simulink model "HCS_Sim_r9_final"  (R2023a)
settings: Solver=ode4  StartTime=0.0  StopTime=24  FixedStep=5e-3  RelTol=1e-3  EnableMultiTasking=on
libraries: simulink x26, simulink_extras x11, arduinolib x8, spspowerguiLib x1
(part 5 of 5)

== matlab function HCS_Sim_r9_final/Total Resource Monitor ==
  data: tou input; grid2fly input; fly2grid input; ev_g2v input; grid2station output; ev_v2g input; station2grid output; opCost output; savings output; ev_g2v_cost output size=[1 3]; ev_v2g_cost output size=[1 3]; grid2fly_cost output; fly2grid_cost output; elec_g2v input; elec_v2g input
function [grid2station, station2grid, opCost, savings, ev_g2v_cost, ev_v2g_cost, grid2fly_cost, fly2grid_cost]   = totalResourceMonitor(tou, grid2fly, fly2grid, ev_g2v, ev_v2g,elec_g2v, elec_v2g)
min = 60; % 1 hr in mins
sec = 60; % 1 min in seconds

ev_g2v_delta = zeros(1, 3);
ev_v2g_delta = zeros(1, 3);
ev_g2v_cost = zeros(1, 3);
ev_v2g_cost = zeros(1, 3);
grid2fly_cost = 0;
fly2grid_cost = 0;

% define rates
if tou == 1
    rate = 0.087; % $/kWh --> $/kWs
elseif tou == 3
    rate = 0.122; % $/kWh --> $/kWs
elseif tou == 4
    rate = 0.182; % $/kWh --> $/kWs
elseif tou == 2
    rate = 0.122; % $/kWh --> $/kWs
else
    rate = 0;
end

% define persistents (memory values)
persistent ev_g2v_prev ev_v2g_prev grid2fly_prev fly2grid_prev grid2station_prev station2grid_prev opCost_prev ...
    savings_prev ev_g2v_cost_prev ev_v2g_cost_prev grid2fly_cost_prev fly2grid_cost_prev total_ev_cost total_ev_cost_prev
if isempty(ev_g2v_prev)
    ev_g2v_prev = zeros(1, 3);
end
if isempty(ev_v2g_prev)
    ev_v2g_prev = zeros(1, 3);
end
if isempty(grid2station_prev)
    grid2station_prev = 0;
end
if isempty(station2grid_prev)
    station2grid_prev = 0;
end
if isempty(opCost_prev)
    opCost_prev = 0;
end
if isempty(savings_prev)
    savings_prev = 0;
end
if isempty(ev_g2v_cost_prev)
    ev_g2v_cost_prev = zeros(1, 3);
end
if isempty(ev_v2g_cost_prev)
    ev_v2g_cost_prev = zeros(1, 3);
end
if isempty(grid2fly_prev)
    grid2fly_prev = 0;
end
if isempty(grid2fly_cost_prev)
    grid2fly_cost_prev = 0;
end
if isempty(fly2grid_prev)
    fly2grid_prev = 0;
end
if isempty(fly2grid_cost_prev)
    fly2grid_cost_prev = 0;
end
if isempty(total_ev_cost)
    total_ev_cost = 0;
end
if isempty(total_ev_cost_prev)
    total_ev_cost_prev = 0;
end

ev_g2v_cost = ev_g2v_cost_prev;
ev_v2g_cost =ev_v2g_cost_prev;


% update kWh I/O counters
grid2station = grid2fly; % init grid2station value with flywheel data first
station2grid = fly2grid; % since the other data is in array format for 1 to
for i = 1:length(ev_g2v) % 3 cars, loop through and sum kWh overall in/out data.
    grid2station = grid2station + ev_g2v(i); % Increment grid2station output by
    station2grid = station2grid + ev_v2g(i); % kWh consumed/discharged by EVs
    
    % compute ev g2v array params (cost, RoC)
    ev_g2v_delta(i) = ev_g2v(i) - ev_g2v_prev(i);
    ev_g2v_cost(i) = ev_g2v_cost_prev(i) + (rate * ev_g2v_delta(i));
    ev_g2v_cost_prev(i) = ev_g2v_cost(i);
    ev_g2v_prev(i) = ev_g2v(i);
    
    % compute ev v2g array params (cost, RoC)
    ev_v2g_delta(i) = ev_v2g(i) - ev_v2g_prev(i);
    ev_v2g_cost(i) = ev_v2g_cost_prev(i) + (rate * ev_v2g_delta(i));
    ev_v2g_cost_prev(i) = ev_v2g_cost(i);
    ev_v2g_prev(i) = ev_v2g(i);

    % total_ev_cost = total_ev_cost_prev + ev_g2v_cost(i);
    % total_ev_cost_prev = total_ev_cost;
end

% compute flywheel params
grid2fly_delta = grid2fly - grid2fly_prev;
grid2fly_cost = grid2fly_cost_prev + (rate * grid2fly_delta);
grid2fly_cost_prev = grid2fly_cost;
grid2fly_prev = grid2fly;

fly2grid_delta = fly2grid - fly2grid_prev;
fly2grid_cost = fly2grid_cost_prev + (rate * fly2grid_delta);
fly2grid_cost_prev = fly2grid_cost;
fly2grid_prev = fly2grid;

% station params
grid2station_delta = grid2station - grid2station_prev; % change in kWh per step
grid2station_prev = grid2station; % save new grid2station state in memory for next pass

station2grid_delta = station2grid - station2grid_prev; % change in kWh per step
station2grid_prev = station2grid; % save new station2grid state in memory for next pass

% calculate total cost of operation
opCost = opCost_prev + (rate * grid2station_delta); % convert to $/kWh
opCost_prev = opCost;
savings = savings_prev + (rate * station2grid_delta);
savings_prev = savings;
% NormalCost = total_ev_cost + elec_g2v;

== matlab function HCS_Sim_r9_final/EV Chargers/EV Charging Function (Revision) ==
  data: time input; ev_soc output; TOU input; EVStart1 input; EVStart2 input; EVStart3 input; EVStop1 input; EVStop2 input; EVStop3 input; scaling input; ev1_soc_init input; ev2_soc_init input; ev3_soc_init input; totC output; totD output; totR output; EV1_state output; EV2_state output; EV3_state output
function [ev_soc, totC, totD, totR, EV1_state, EV2_state, EV3_state] = ev_chg_current(time, TOU, EVStart1, EVStart2, EVStart3, EVStop1, EVStop2, ...
    EVStop3, scaling, ev1_soc_init, ev2_soc_init, ev3_soc_init)
% TIME OF USE INTEGERS
% [1] off peak
% [2] mid peak low/down
% [3] mid peak high
% [4] on peak
% [5] null


% (!!!) SCALING VALUE (!!!)
socScalar = 0.00055;      %
% -------------------------

ev_soc_init = 0.01 * [ev1_soc_init , ev2_soc_init, ev3_soc_init];
persistent EVSOC_Array ev_soc_prev
if isempty(EVSOC_Array)
    EVSOC_Array = zeros(1, 3);
end

if isempty(ev_soc_prev)
    ev_soc_prev = zeros(1, 3);
end

for j = 1:length(ev_soc_prev)
    if ev_soc_prev(j) == 0
    ev_soc_prev(j) = ev_soc_prev(j) + ev_soc_init(j);
    end
end



persistent TotC_Array TotC_Array_prev TotDe_Array TotDe_Array_prev TotRe_Array TotRe_Array_prev
if isempty(TotC_Array)
    TotC_Array = zeros(1, 3);
end
if isempty(TotC_Array_prev)
    TotC_Array_prev = zeros(1, 3);
end
if isempty(TotDe_Array)
    TotDe_Array = zeros(1, 3);
end
if isempty(TotDe_Array_prev)
    TotDe_Array_prev = zeros(1, 3);
end
if isempty(TotRe_Array)
    TotRe_Array = zeros(1, 3);
end
if isempty(TotRe_Array_prev)
    TotRe_Array_prev = zeros(1, 3);
end

persistent initAdded
if isempty(initAdded)
    initAdded = zeros(1, 3); % Flags to check if initial SoC has been added
end

persistent EVT_Array
if isempty(EVT_Array)
    EVT_Array = zeros(1, 3);
end

%initializes at 0
%this goes high when done charging
persistent charge
if isempty(charge)
    charge = zeros(1, 3);
end

%goes high when discharged
persistent discharge
if isempty(discharge)
    discharge = zeros(1, 3);
end

%TOU when  the car finishes charging
persistent endCHARGE
if isempty(endCHARGE)
    endCHARGE = zeros(1, 3);
end
%TOU when car finishes discharging
persistent endDISCHARGE
if isempty(endDISCHARGE)
    endDISCHARGE = zeros(1, 3);
end

EVStartArray = [EVStart1, EVStart2, EVStart3];
EVStopArray = [EVStop1 + EVStart1, EVStop2 + EVStart2, EVStop3 + EVStart3];

% this chunk simply adds an initial SoC depending on the defined initial
% SoC (per EV)
for k = 1:length(ev_soc_prev)
    if time >= ev_soc_prev(k) && ~initAdded(k)
        ev_soc_prev(k) = ev_soc_prev(k);
        initAdded(k) = 1; % Set the flag so it doesn't add init SoC again
    elseif time < EVStartArray(k) && ~initAdded(k)
        ev_soc_prev(k) = 0;
    elseif time > EVStopArray(k)
        ev_soc_prev(k) = 0;
    end
end



% charges car
% Loop through cars 1, 2 and 3
for i = 1:length(EVStartArray)

    if time >= EVStartArray(i) && time <= EVStopArray(i)
        EVT_Array(i) = 1;
    else
        EVT_Array(i) = 0; 
    end

    if EVT_Array(i) == 1  % if EV is connected, then
        if (ev_soc_prev(i) < 1 && ev_soc_prev(i) <= 0.999) && charge(i) == 0
            EVSOC_Array(i) = ev_soc_prev(i) + (socScalar * scaling);
            TotC_Array(i) = TotC_Array_prev(i) + (socScalar * scaling); % total % SoC from station2ev
            endCHARGE(i) = -1; % -1 value to indicate that charging has NOT completed
        elseif (ev_soc_prev(i) <= 1 && ev_soc_prev(i) > 0.999) && charge(i) == 0
            EVSOC_Array(i) = ev_soc_prev(i) + (1 - ev_soc_prev(i));
            TotC_Array(i) = TotC_Array_prev(i) + (1 - ev_soc_prev(i)); % Add charge to tracked total
            charge(i) = 1; % set charge flag == 1 when close to 100% charged
        elseif (ev_soc_prev(i) <= 1 && ev_soc_prev(i) > 0.999) && charge(i) == 1
            EVSOC_Array(i) = ev_soc_prev(i) + (1 - ev_soc_prev(i));
            TotC_Array(i) = TotC_Array_prev(i) + (1 - ev_soc_prev(i));
            endCHARGE(i) = TOU; % after EV confirmed completed charging, endCHARGE logs TOU when charge completed
        end

        if endCHARGE(i) ~= -1 % if charging HAS completed
            endDISCHARGE(i) = -1;
            if ((TOU == 4 || TOU > endCHARGE(i)) && ev_soc_prev(i) > 0.90) && endDISCHARGE(i) == -1
                EVSOC_Array(i) = ev_soc_prev(i) - (socScalar * scaling);
                TotDe_Array(i) = TotDe_Array_prev(i) + (socScalar * scaling);
                if EVSOC_Array(i) <= 0.9
                    endCHARGE(i) = -1;
                    endDISCHARGE(i) = TOU;
                else
                    endDISCHARGE(i) = -1; % endDISCHARGE flag == -1, discharging has NOT completed
                end
            end
        end
    
        if endDISCHARGE(i) ~= -1 % if discharging HAS completed
            if TOU < endDISCHARGE(i) && TOU ~= 4
                if (ev_soc_prev(i) < 1 && ev_soc_prev(i) <= 0.999)
                    EVSOC_Array(i) = ev_soc_prev(i) + (socScalar * scaling); % total SoC including init %
                    TotC_Array(i) = TotC_Array_prev(i) + (socScalar * scaling); % total % SoC from station2ev
                    TotRe_Array(i) = TotRe_Array_prev(i) + (socScalar * scaling); % total % SoC from station2ev
                    endCHARGE(i) = -1;
                elseif (ev_soc_prev(i) <= 1 && ev_soc_prev(i) > 0.999)
                    EVSOC_Array(i) = ev_soc_prev(i) + (1 - ev_soc_prev(i)); % drastically reduce charge rate
                    TotC_Array(i) = TotC_Array_prev(i) + (1 - ev_soc_prev(i)); % Add charge to tracked total
                    TotRe_Array(i) = TotRe_Array_prev(i) + (1 - ev_soc_prev(i));
                    endCHARGE(i) = TOU;
                    endDISCHARGE(i) = -1;
                end
            elseif TOU < endDISCHARGE(i) && TOU == 4
                if (ev_soc_prev(i) < 1 && ev_soc_prev(i) <= 0.999)
                    EVSOC_Array(i) = ev_soc_prev(i) + (0.00025 * scaling); % slow down charge rate
                    TotC_Array(i) = TotC_Array_prev(i) + (0.00025 * scaling); % total % SoC from station2ev
                    endCHARGE(i) = -1;
                elseif (ev_soc_prev(i) <= 1 && ev_soc_prev(i) > 0.999)
                    EVSOC_Array(i) = ev_soc_prev(i) + (1 - ev_soc_prev(i)); % drastically reduce charge rate
                    TotC_Array(i) = TotC_Array_prev(i) + (1 - ev_soc_prev(i)); % Add charge to tracked total
                    endCHARGE(i) = TOU;
                    endDISCHARGE(i) = -1;
                end
            end
        end
    else
        EVSOC_Array(i) = 0;
    end
    ev_soc_prev(i) = EVSOC_Array(i);
    TotC_Array_prev(i) = TotC_Array(i);
    TotDe_Array_prev(i) = TotDe_Array(i);
    TotRe_Array_prev(i) = TotRe_Array(i);
end


ev_soc = EVSOC_Array;

totC = TotC_Array;
totD = TotDe_Array;
totR = TotRe_Array;

EV1_state = EVT_Array(1); % EV connection statuses
EV2_state = EVT_Array(2);
EV3_state = EVT_Array(3);

== matlab function HCS_Sim_r9_final/Subsystem1/HighPressure ==
  data: concost output; H70exp input; FCEVCheck input; H70Tank output; CurH70 output; counter1 output; counter2 output; condenserOn output; tou input; scaling input
function [concost, H70Tank,CurH70,counter1,counter2,condenserOn]= fcn(H70exp,FCEVCheck, tou, scaling)
%CUR h70 is the initial cond + expense + income from h20
%h70tank is the expense offset with the 5kg initial condition
%condenser and pressurize placeholders, unused
%counter 1 used to calculate total H20 needed for the H70 exp
%H70exp is the total expense of h70 used by FCEVS
%FCEV check goes high when the sim time matches the start time for an FCEV


%initializes at 0
persistent H70tot
if isempty(H70tot)
    H70tot = 0;
end
persistent counter
persistent count1
persistent count2
persistent count3
persistent count4
if isempty(counter)
    counter = 0;
    count1 = 0;
    count2 = 0;
    count3 = 0;
    count4 = 0;
end


%updates h70 with new expense only when FCEV is present
if  FCEVCheck == 1
    H70tot =+ H70exp;
else
     H70tot = H70tot + 0;
     % pause(1);
end

%adds 5kg inital condition as offset
%Cur H70 keeps track of current h70 with all expense and income
H70Tank = H70tot +5 *scaling;
CurH70 = H70exp + 5 + 0.1*counter*scaling;

%counter is tally of H20 being pressurized and added to this tank
if CurH70 < 10
    counter = counter +0.125;
    %pause(10);
    % pressurize = 1;
 if tou == 1
     rate = 0.087;
    count1 = count1 +0.125*scaling*rate;
 elseif tou == 2
     rate = 0.122;
     count2 = count2 +0.125*scaling*rate;
 elseif tou == 3
     rate = 0.122;
     count3 = count3 +0.125*scaling*rate;
 elseif tou == 4
     rate = 0.182;
     count4 = count4 +0.125*scaling*rate;
 else
     rate = 0;
 end
    
end
%these are multipliers that can be adjusted to effect the electrolysis rate
    counter1 = 0.1*counter*scaling;
    counter2 = ((scaling * counter1-10)/2)+5;
    % pressurize = 0;
 rate = 0;

    
 %below here is all unused   
 if CurH70 == 10
       condenserOn = 0;
 else
     condenserOn = 1;
 end

%setting KWH for condensing for kg of h2
conpow = 0.136;
persistent concost_prev
if isempty (concost_prev)
    concost_prev = 0;
end
 concost = (count1 + count2 +count3 + count4)*conpow;
 concost_prev = concost;

== matlab function HCS_Sim_r9_final/Subsystem1/LowPressure ==
  data: presout output; H20exp input; TOU input; elecout1 output; HydrolIn1 output; H20Tank1 output; ElecInHydOut output; hydInElecOut output; scaling input; ElecCost output; RevElecCost output
function [presout, elecout1, HydrolIn1,H20Tank1, ElecInHydOut, hydInElecOut, ElecCost, RevElecCost]= fcn(H20exp, TOU,scaling)
%h20exp is the total expense of h20 going to h70 thru condenser
%Tou is TOU
%

ElecInHydOut = 0;
hydInElecOut = 0;
presout = 0;
%%initializing persistent
persistent elecout
if isempty(elecout)
    elecout = 0;
end

persistent HydrolIn
if isempty(HydrolIn)
    HydrolIn = 0;
end

persistent H20Tank
if isempty(H20Tank)
    H20Tank = 0;
end

% if H20Tank > 0
    H20Tank = (HydrolIn - H20exp - elecout) *scaling + 5;

% else
%     H20Tank = HydrolIn - H20exp - elecout
%replenish Hydrogren if below buffer discharge if above based off peak
%demand
persistent eleccount1
persistent reveleccount1
persistent eleccount2
persistent reveleccount2
persistent eleccount3
persistent reveleccount3 
persistent eleccount4
persistent reveleccount4
persistent eleccountT
persistent reveleccountT
if isempty(eleccount1)
    eleccount1 = 0;
    reveleccount1 = 0;
    eleccount2 = 0;
    reveleccount2 = 0;
    eleccount3 = 0;
    reveleccount3 = 0;
    eleccount4 = 0;
    reveleccount4 = 0;
    eleccountT = 0;
    reveleccountT = 0;
end

if TOU == 1
    if H20Tank <= 5
        HydrolIn = HydrolIn + 0.01*scaling;
        elecout = elecout;
        ElecInHydOut = 1;

        eleccount1 = eleccount1 +(0.01*scaling)*53*0.087;
    elseif H20Tank > 5.2
        elecout = elecout +0.003*scaling;
        HydrolIn = HydrolIn;
        ElecInHydOut = 0;
        hydInElecOut = 1;
        reveleccount1 = reveleccount1 + (0.003*scaling)*33.6*0.087;
    else
        HydrolIn = HydrolIn;
        elecout = elecout;
        ElecInHydOut = 0;
        eleccount1 = eleccount1;
        reveleccount1 = reveleccount1;
    end
elseif TOU == 2
    if H20Tank <= 7
        HydrolIn = HydrolIn + 0.01*scaling;
        elecout = elecout;
        ElecInHydOut = 1;

        eleccount2 = eleccount2 +(0.01*scaling)*53*0.122;
    elseif H20Tank > 7.2
        elecout = elecout +0.003*scaling;
        HydrolIn = HydrolIn;
        ElecInHydOut = 0;
        reveleccount2 = reveleccount2 + (0.003*scaling)*33.6*0.122;
        hydInElecOut = 1;
    else
        HydrolIn = HydrolIn;
        elecout = elecout;
        ElecInHydOut = 0;
        eleccount2 = eleccount2;
        reveleccount2 = reveleccount2;
    end
elseif TOU == 3
    if H20Tank <= 7
        HydrolIn = HydrolIn + 0.01*scaling;
        elecout = elecout;
        ElecInHydOut = 1;
        
        eleccount3 = eleccount3 +(0.01*scaling)*53*0.122;
    elseif H20Tank > 7.2
        elecout = elecout +0.003*scaling;
        HydrolIn = HydrolIn;
        ElecInHydOut = 0;
        hydInElecOut = 1;
        reveleccount3 = reveleccount3 + (0.003*scaling)*33.6*0.122;
    else
        HydrolIn = HydrolIn;
        elecout = elecout;
        ElecInHydOut = 0;
        eleccount3 = eleccount3;
        reveleccount3 = reveleccount3;
    end
elseif TOU == 4
    if H20Tank <= 9
        HydrolIn = HydrolIn + 0.01*scaling;
        elecout = elecout;
        ElecInHydOut = 1;

        eleccount4 = eleccount4 +(0.01*scaling)*53*0.182;
    elseif H20Tank > 9.2
        elecout = elecout +0.003*scaling;
        HydrolIn = HydrolIn;
        ElecInHydOut = 0;
        hydInElecOut = 1;
        reveleccount4 = reveleccount4 + (0.003*scaling)*33.6*0.182;
    else
        HydrolIn = HydrolIn;
        elecout = elecout;
        ElecInHydOut = 0; 
        eleccount4 = eleccount4;
        reveleccount4 = reveleccount4;
    end
else
    % HydrolIn = HydrolIn;
    % elecout = elecout;
    % eleccountT = eleccount1 + eleccount2 + eleccount3 + eleccount4
    % reveleccountT = reveleccount1 + reveleccount2 +reveleccount3 +reveleccount4
    
end
persistent reveleccountprev
persistent eleccountprev
if isempty (reveleccountprev)
    reveleccountprev = 0;
    eleccountprev = 0;
end
% reveleccount1
% reveleccount2
% reveleccount3
% reveleccount4
eleccountT = eleccount1 + eleccount2 + eleccount3 + eleccount4;
reveleccountT = reveleccount1 + reveleccount2 +reveleccount3 +reveleccount4;
eleccountprev = eleccountT;
reveleccountprev = reveleccountT;
ElecCost = eleccountT;
RevElecCost = reveleccountT;
% ElecInHydOut = 0;
elecout1 = elecout;
HydrolIn1 = HydrolIn;
H20Tank1 = H20Tank;

% if H20Tank <= 5 && TOU == 1   
%     HydrolIn = HydrolIn + 0.01*scaling;
%     elecout = elecout;
%     ElecInHydOut = 1;
% elseif H20Tank <= 7 && TOU == 3
% elseif H20Tank <= 9 && TOU == 4
% elseif H20Tank <= 7 && TOU == 2
% 
% 
% 
% 
% else 
%     elecout = elecout +0.003*scaling;
%     HydrolIn = HydrolIn;
%     ElecInHydOut = 0;
%     TOU;
% 
% 
% end
% elecout1 = elecout;
% HydrolIn1 = HydrolIn;
% H20Tank1 = H20Tank;





% persistent wait
% if isempty(wait)
%    wait = 0;
% end
% % if isempty(presout)
% %    presout = 0;
% % end
% if callpres == 1
%    presout = 1;
%     % if wait == 0
%    %     % H35 =-
%    %     presout = 1;
%    %     wait = 1;
%    % 
%    %  else
%    %      % pause(1);
%    %      wait = 0;
%    %      presout = 0;
%    % end
% else
%     presout = 0;
% end

%if h tank < 5 AND TOU = off peak || h tank < 7 AND tou = mid (up) high ||
%h tank < 9 AND tou = on peak || h tank < 7 AND tou = mid (down) low

== matlab function HCS_Sim_r9_final/Subsystem1/MATLAB Function ==
  data: FCEVIn input; FCEVPres output
function FCEVPres = fcn(FCEVIn)
Counter = 0;
if FCEVIn == 1
    while Counter < 20
        FCEVPres = 1;
        Counter = Counter + 1
    end
    FCEVPres = 0;
end
FCEVPres =0;

== matlab function HCS_Sim_r9_final/Subsystem1/MATLAB Function1 ==
  data: time input; fcev1 input; fcev2 input; fcev3 input; fcev4 input; fcev5 input; y1 output; y2 output; y3 output; y4 output; y5 output; stat1 input; stat2 input; stat3 input; stat4 input; stat5 input
function [y1, y2, y3, y4, y5] = fcn(time,fcev1, fcev2, fcev3, fcev4,  fcev5, stat1, stat2, stat3, stat4, stat5)
%persistent values y1y to hold status for charging

persistent y1y
if isempty(y1y)
    y1y = 0;
end
persistent y2y
if isempty(y2y)
    y2y = 0;
end
persistent y3y
if isempty(y3y)
    y3y = 0;
end
persistent y4y
if isempty(y4y)
    y4y = 0;
end
persistent y5y
if isempty(y5y)
    y5y = 0;
end
%time > (fcev1 -0.5 ) && time < (fcev1 + 0.5) && stat1 == 1
%time == fcev1 && stat1 == 1

%setting y1y based of user inputs (is the car plugged in)
if time > (fcev1 -0.005 ) && time < (fcev1 + 0.005) && stat1 == 1
    if y1y ~= 1
        y1y = 1;
     
    end
else
    y1y = 0;
end

if time > (fcev2 -0.005 ) && time < (fcev2 + 0.005) && stat2 == 1
    if y2y ~= 1
        y2y = 1;
     
    end
else
    y2y = 0;
end

if time > (fcev3 -0.005 ) && time < (fcev3 + 0.005) && stat3 == 1
    if y3y ~= 1
        y3y = 1;
     
    end
else
    y3y = 0;
end
if time > (fcev4 -0.005 ) && time < (fcev4 + 0.005) && stat4 == 1
    if y4y ~= 1
        y4y = 1;
     
    end
else
    y4y = 0;
end

if time > (fcev5 -0.005 ) && time < (fcev5 + 0.005) && stat5 == 1
    if y5y ~= 1
        y5y = 1;
     
    end
else
    y5y = 0;
end

y1 =y1y;
y2= y2y;
y3 = y3y;
y4= y4y;
y5 = y5y;

== matlab function HCS_Sim_r9_final/Subsystem1/MATLAB Function2 ==
  data: concost input; H2Expense output; electrolcost input; reveleccost input; H2Payback output
function [H2Expense, H2Payback] = fcn(concost, electrolcost, reveleccost)

H2Expense = concost + electrolcost;
H2Payback =reveleccost;

== matlab function HCS_Sim_r9_final/Subsystem1/Total Usage ==
  data: Time input; H2Out output; Done1 output; Done2 output; Done3 output; Done4 output; Done5 output; H70Out output; H2Feedback input; FT1 input; FT2 input; FT3 input; FT4 input; FT5 input; FSOC1 input; FSOC2 input; FSOC3 input; FSOC4 input; FSOC5 input; H70Bar input
function [H2Out,Done1,Done2,Done3,Done4, Done5, H70Out] = fcn(Time, H2Feedback, FT1, FT2, FT3, FT4, FT5, FSOC1, FSOC2, FSOC3, FSOC4, FSOC5,H70Bar)
%H2out / H70out feedback for H2 cost
%Done are feedback to tell previous block that FCEV is full charge
%FTs is boolean status for if the car is there
%SOC is the charge set at dashboard
%H2out and H70 bar are both feedback for total hyd cost
%time unused in this block


Done1 = 0;
Done2 = 0;
Done3 = 0;
Done4 = 0;
Done5 = 0;
%H70Bar = 5;
%if Time == 5
%    H70Out = 5
%end
%if Init == 0
%    H70Bar = 5;
%    InitOut = 1;
%else
 %   H70Out = H70Bar;
%end
%InitOut = 1;

%these blocks check for the FCEV and subtract the KG from the h70 tank
%needed to fill them to 5kg
if FT1 == true
    H2Out = H2Feedback + (5 - FSOC1);
    H70Bar = H70Bar - (5 - FSOC1);
    %H70Fin = H70Fin -H70Bar
    Done1 = 1;
    %InitOut = 1;
     
elseif FT2 == true
    H2Out = H2Feedback + (5 - FSOC2);
    H70Bar = H70Bar - (5 - FSOC2);
    %H70Fin = H70Fin -H70Bar
    Done2 = 1;
    %InitOut = 1;
elseif FT3 == true
    H2Out = H2Feedback + (5 - FSOC3);
    H70Bar = H70Bar - (5 - FSOC3);
   % H70Fin = H70Fin -H70Bar
    Done3 = 1;
    %InitOut = 1;
elseif FT4 == true
    H2Out = H2Feedback + (5 - FSOC4);
    H70Bar = H70Bar - (5 - FSOC4);
  %  H70Fin = H70Fin -H70Bar
    Done4 = 1;
    %InitOut = 0;
elseif FT5 == true
    H2Out = H2Feedback + (5 - FSOC5);
    H70Bar = H70Bar - (5 - FSOC5);
    %H70Fin = H70Fin -H70Bar
    Done5 = 1;
   % InitOut = 1;
else
    H2Out = (H2Feedback +0);
    
end
H70Out = H70Bar;

== matlab function HCS_Sim_r9_final/TOU converter ==
  data: Low input; TOU output; MidU input; High input; MD input
function TOU = fcn(Low,MidU,High,MD)

if Low == 1
    TOU = 0;
elseif MidU == 1
    TOU = 1;
elseif High == 1
    TOU = 2;
elseif MD == 1
    TOU = 3;
else
    TOU = 4;
end

== matlab function HCS_Sim_r9_final/MATLAB Function3 ==
  data: tou input; duty output
function duty = int_2_pwm(tou)

if tou == 1 
    duty = 0.10;
elseif tou == 2 % mid peak low
    duty = 0.30;
elseif tou == 3 % mid peak high
    duty = 0.50;
elseif tou == 4
    duty = 0.70;
elseif tou == 5
    duty = 0.90;
else
    duty = 1.0;
end

duty = duty * 255;

== matlab function HCS_Sim_r9_final/EV Chargers/SoC-kWh Conversion (EVs) ==
  data: totC input; kwh_g2v output; totD input; totR input; kwh_v2g output
function [kwh_g2v, kwh_v2g] = soc_kwh_convert(totC, totD, totR)
% Function purpose is to take EV SoC and compute kWh consumed
% kwh_g2v output is a 1x3 array logging kWh drawn from the grid
% kwh_v2g output is 1x3 array logging kWh sold back to grid
ev_battery_capacity = 65; % kWh (full battery capacity)

totC_Array = totC;
totD_Array = totD;
totR_Array = totR;
kwh_g2v = zeros(1, 3);
kwh_v2g = zeros(1, 3);

for i = 1:length(totC_Array)
    kwh_g2v(i) = ev_battery_capacity * (totC_Array(i) + totR_Array(i));
    kwh_v2g(i) = ev_battery_capacity * totD_Array(i);
end

== matlab function HCS_Sim_r9_final/MATLAB Function1 ==
  data: tou input; on_peak output; off_peak output; mid_peak_lo output; mid_peak_hi output; null output
function [on_peak, off_peak, mid_peak_lo, mid_peak_hi, null] = tou_translate(tou)

if tou == 0
    on_peak = logical(false);
    off_peak = logical(false);
    mid_peak_lo = logical(false);
    mid_peak_hi = logical(false);
    null = logical(true);
elseif tou == 1
    on_peak = logical(false);
    off_peak = logical(true);
    mid_peak_lo = logical(false);
    mid_peak_hi = logical(false);
    null = logical(false);
elseif tou == 2
    on_peak = logical(false);
    off_peak = logical(false);
    mid_peak_lo = logical(true);
    mid_peak_hi = logical(false);
    null = logical(false);
elseif tou == 3
    on_peak = logical(false);
    off_peak = logical(false);
    mid_peak_lo = logical(false);
    mid_peak_hi = logical(true);
    null = logical(false);
elseif tou == 4
    on_peak = logical(true);
    off_peak = logical(false);
    mid_peak_lo = logical(false);
    mid_peak_hi = logical(false);
    null = logical(false);
else
    on_peak = logical(false);
    off_peak = logical(false);
    mid_peak_lo = logical(false);
    mid_peak_hi = logical(false);
    null = logical(true);
end

end

== matlab function HCS_Sim_r9_final/MATLAB Function ==
  data: clock input; time output; smplTime input; dt output; tou output; simTime input; simLength input; szn input; days input; tou_int output; scalingFactor output; dashscaling output
function [time, dt, tou, tou_int, scalingFactor, dashscaling] = fcn(clock, smplTime, simTime, simLength, szn, days)
    % Adjusted simulation time to span over 'days' days
    % First, calculate the total simulation time in hours for the given number of days
    totalSimHours = simLength * days;
    
    % Convert clock (in seconds) to actual simulation time (in hours)
    % Instead of scaling the entire simulation to fit within a single day,
    % scale it based on the total simulation hours specified by 'days'
    scalingFactor = totalSimHours / (simTime / 3600);
    scaledTime = (clock / 3600) * scalingFactor; % Convert clock to hours and scale based on totalSimHours
    %dashscaling = 3600 / scalingFactor
    dashscaling = scalingFactor / 3600;
    tou = "null";
    tou_int = 0;

    % Outputs
    time = scaledTime; % The scaled simulation time in hours, adjusted for multiple days
    dt = (smplTime / simTime) * smplTime * time; % The timestep in hours

    % Determine the time of use (TOU) state based on the scaled simulation time
    % For TOU calculations, use mod(time, 24) to determine the time of day for TOU state decisions
    currentTimeOfDay = mod(time, 24);

    % Assuming the 'hrs' variable represents an hour in the context of currentTimeOfDay
    hrs = 1; % 1 hour in terms of scaled simulation time

    % Update TOU state checks to use currentTimeOfDay for daily cycle logic
    if szn == 0
        if (currentTimeOfDay >= 0*hrs && currentTimeOfDay <= 7*hrs) || (currentTimeOfDay > 19*hrs && currentTimeOfDay <= 24*hrs)
            tou = "off_peak";
            tou_int = 1; % off peak
        elseif (currentTimeOfDay > 7*hrs && currentTimeOfDay <= 11*hrs)
            tou = "mid_peak_hi";
            tou_int = 3; % mid peak hi
        elseif (currentTimeOfDay > 11*hrs && currentTimeOfDay <= 17*hrs)
            tou = "on_peak";
            tou_int = 4; % on peak
        elseif (currentTimeOfDay > 17*hrs && currentTimeOfDay <= 19*hrs)
            tou = "mid_peak_lo";
            tou_int = 2; % mid peak lo
        else
            tou = "null";
            tou_int = 0; % null/error
        end
    elseif szn == 1
        if (currentTimeOfDay >= 0*hrs && currentTimeOfDay <= 7*hrs) || (currentTimeOfDay > 19*hrs && currentTimeOfDay <= 24*hrs)
            tou = "off_peak";
            tou_int = 1; % off peak
        elseif (currentTimeOfDay > 7*hrs && currentTimeOfDay <= 11*hrs)
            tou = "on_peak";
            tou_int = 4; % on peak
        elseif (currentTimeOfDay > 11*hrs && currentTimeOfDay <= 17*hrs)
            tou = "mid_peak_lo";
            tou_int = 2; % mid peak lo
        elseif (currentTimeOfDay > 17*hrs && currentTimeOfDay <= 19*hrs)
            tou = "on_peak";
            tou_int = 4; % on peak
        else
            tou = "null";
        end
    end 
end

== matlab function HCS_Sim_r9_final/EV Chargers/MATLAB Function3 ==
  data: ev_start_signal input; bilat_OK input; chargeEnable output; tou_int input; bilatEnable output; maxCharge input; incrementEV output
function [chargeEnable, bilatEnable, incrementEV] = ev_charge_ctrl(ev_start_signal, bilat_OK, tou_int, maxCharge)
    s = 0;
    bilatEnable = 0;
    chargeEnable = 0;
    
    % loop only starts if TOU is ON PEAK and if an EV has been detected by
    % the EVSE
    while (tou_int == 4 && ev_start_signal == 1)
        if bilat_OK == 1
            bilatEnable = 1; % bilateral discharge enabled
        else
            bilatEnable = 0; % bilateral discharge disabled
        end
        
        if (ev_start_signal == 1) && (bilat_OK == 0)
            chargeEnable = 1; % car is connected and battery is > 90% charged AND more then 2% of total capacity is available
        else
            chargeEnable = 0;
        end
    end
    
    % if bilat_OK == 0 (EV not ready for V2G) the vehicle is OK to charge
    % but is not currently, enable charging
    if (chargeEnable == 0) && (bilatEnable == 0)
        chargeEnable = 1;
    end

    % if bilateral charging is OFF and battery is NOT at max capacity, increment the EV
    % charge 
    if bilatEnable == 0 && maxCharge == 1
        incrementEV = 1; % increment charge
    else
        incrementEV = 0;
    end

    % if (chargeEnable == 1 && bilatEnable == 0) && maxCharge == 1
    %     rechargeTrig = 1; % send signal to controller to switch from Off/Bidirectional state to recharge mode
    % else
    %     rechargeTrig = 0;
    % end
    % 

end
